simulink model "Projecto"  (R2018a)
settings: Solver=ode4  StartTime=0.0  StopTime=2  FixedStep=5e-6  RelTol=1e-3
values from neighbouring files (symbols this model uses):
  fn = 60    [parametros_motor.m]
  J = 0.089    [parametros_motor.m]
  Llr = 0.002    [parametros_motor.m]
  Lls = 0.002    [parametros_motor.m]
  Pn = 2130    [parametros_motor.m]
  pp = 2    [parametros_motor.m]
  ref_flux = 0.6    [parametros_motor.m]
  ref_vel = 500    [parametros_motor.m]
  Rr = 0.816    [parametros_motor.m]
  Rs = 0.435    [parametros_motor.m]
  Tload = 10    [parametros_motor.m]
  Vdc = 500    [parametros_motor.m]
  Vn = 220    [parametros_motor.m]
undefined symbols (not defined in the file or in its folder): gcbh, pe_sli_rtmsupport
libraries: powerlib x12, powerlib_meascontrol x4, fuzblock x1, spsDrivesSpeedControllerModel x1
settings Model: Creator=up201604509  LastModifiedBy=up201604509
settings SolverCC: ZeroCrossAlgorithm=Adaptive  AlgebraicLoopSolver=LineSearch
settings DebuggingCC: AlgebraicLoopMsg=none  MaxConsecutiveZCsMsg=none

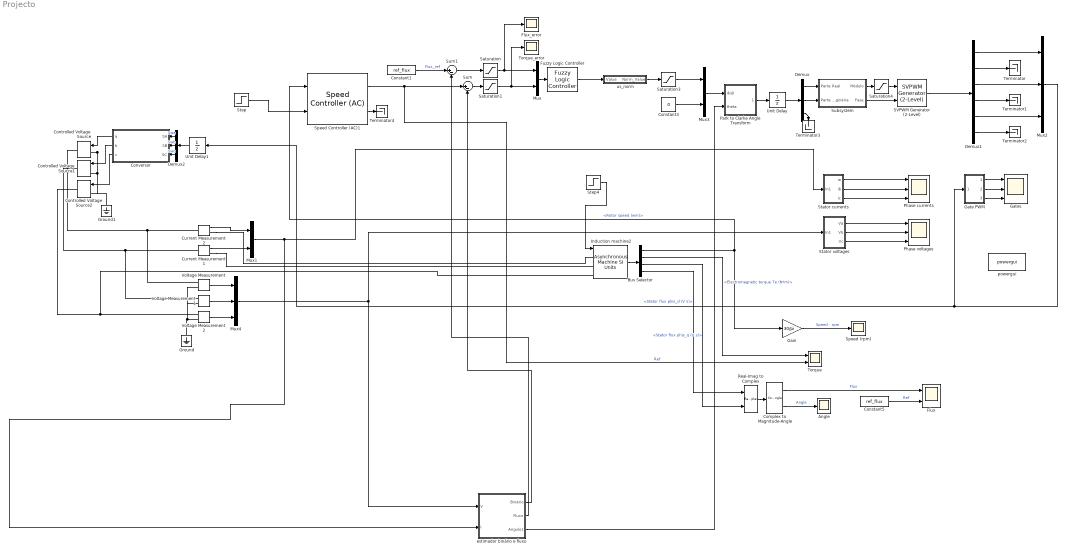
== system Projecto ==
  Angle : Scope
  Bus Selector : BusSelector  OutputSignals=Mechanical.Rotor speed (wm),Mechanical.Electromagnetic torque Te (N*m),Stator measurements.Stator flux phis_q (V s),Stator measurements.Stator flux phis_d (V s)
  Complex to Magnitude-Angle : ComplexToMagnitudeAngle
  Constant1 : Constant  Value=ref_flux
  Constant3 : Constant  Value=0
  Constant5 : Constant  Value=ref_flux
  Controlled Voltage Source : powerlib/Electrical Sources/Controlled Voltage Source  Initialize=on  Source_Type=AC  Amplitude=0  Phase=0  Frequency=0  Measurements=Voltage
      settings: SourceProductName=Simscape Electrical
  Controlled Voltage Source1 : powerlib/Electrical Sources/Controlled Voltage Source  Initialize=on  Source_Type=AC  Amplitude=0  Phase=0  Frequency=0  Measurements=Voltage
      settings: SourceProductName=Simscape Electrical
  Controlled Voltage Source2 : powerlib/Electrical Sources/Controlled Voltage Source  Initialize=on  Source_Type=AC  Amplitude=0  Phase=0  Frequency=0  Measurements=Voltage
      settings: SourceProductName=Simscape Electrical
  Conversor : Subsystem
  Current Measurement1 : powerlib/Measurements/Current Measurement  Tag=PoWeRsYsTeMmEaSuReMeNt  PhasorSimulation=off  OutputType=Complex  PSBequivalent=0
      settings: SourceProductName=Simscape Electrical
  Current Measurement2 : powerlib/Measurements/Current Measurement  Tag=PoWeRsYsTeMmEaSuReMeNt  PhasorSimulation=off  OutputType=Complex  PSBequivalent=0
      settings: SourceProductName=Simscape Electrical
  Demux : Demux  Outputs=3
  Demux1 : Demux  Outputs=6
  Demux2 : Demux  Outputs=3
  Flux : Scope  NumInputPorts=2
  Flux_error : Scope
  Fuzzy Logic Controller : fuzblock/Fuzzy Logic  Controller  FIS=controler  OutputSampleNumber=101  DataType=double  FuzzifiedInputs=off  RuleFiringStrengths=off  RuleOutputs=off  AggregatedOutputs=off  SimulateUsing=Interpreted execution  OutOfRangeInputValueMessage=warning  NoRuleFiredMessage=warning  EmptyOutputFuzzySetMessage=warning
  Gain : Gain  Gain=30/pi  SaturateOnIntegerOverflow=on  OutDataTypeStr=Inherit: Same as input  ParamDataTypeStr=Inherit: Same as input
  Gate PWM : Subsystem
  Gates : Scope  NumInputPorts=3
  Ground : powerlib/Elements/Ground  LConnTagsString=a
      settings: SourceProductName=Simscape Electrical
  Ground1 : powerlib/Elements/Ground  LConnTagsString=a
      settings: SourceProductName=Simscape Electrical
  Induction machine2 : powerlib/Machines/Asynchronous Machine SI Units  RotorType=Squirrel-cage  PresetModel=No  MechanicalLoad=Torque Tm  ShowDetailedParameters=on  ReferenceFrame=Stationary  Units=SI  MeasurementBus=off  NominalParameters="[Pn  Vn  fn]"  Stator=[Rs Lls]  Rotor=[Rr Llr]  Cage1=[ 0.022 0.226/377]  Cage2=[ 0.022 0.226/377]  Lm=Lm  Mechanical="[J  0.001 pp]"  PolePairs=2  InitialConditions=[1 0 0 0 0 0 -120 120]  SimulateSaturation=off  Saturation=[0 0;0 0]  LoadFlowParameters=0  TsPowergui=0  TsBlock=-1  IterativeModel=Trapezoidal non iterative  IterativeDiscreteModel=Trapezoidal non iterative  Pmec=0
      settings: SourceProductName=Simscape Electrical
  Mux : Mux  Inputs=2
  Mux1 : Mux  Inputs=2
  Mux2 : Mux  Inputs=3
  Mux3 : Mux  Inputs=2
  Mux4 : Mux  Inputs=3
  Park to Clarke Angle Transform : Subsystem  AncestorBlock=peTransforms/Park to Clarke Angle Transform  LoadFcn=pe_sli_rtmsupport( 'loadfcn', gcbh );  mask(Park to Clarke Angle Transform){AxisAlignment=D-axis}
      mask prompts: AxisAlignment "Phase-a axis alignment:"
      mask help: This block implements an angle transformation from Park coordinates to Clarke coordinates.
      mask init:
      | switch AxisAlignment
      |     case 'Q-axis'
      |         Offset = pi/2;
      |     case 'D-axis'
      |         Offset = 0;
      |     otherwise
      | end
      settings: CopyFcn=pe_sli_rtmsupport( 'copyfcn', gcbh );  DeleteFcn=pe_sli_rtmsupport( 'deletefcn', gcbh );  ModelCloseFcn=pe_sli_rtmsupport( 'modelclosefcn', gcbh );  PostSaveFcn=pe_sli_rtmsupport( 'postsavefcn', gcbh );  PreCopyFcn=pe_sli_rtmsupport( 'precopyfcn', gcbh );  OpenFcn=pe_sli_rtmsupport( 'openfcn', gcbh );  CloseFcn=pe_sli_rtmsupport( 'closefcn', gcbh );  PreDeleteFcn=pe_sli_rtmsupport( 'predeletefcn', gcbh );
      mask Help: web(nesl_help(gcbh))
      mask TypeOptions AxisAlignment: Q-axis | D-axis
      mask Display: pe.mask.drawParkToClarkeAngleTransform();
  Phase currents : Scope  NumInputPorts=3
  Phase voltages : Scope  NumInputPorts=3
  Real-Imag to Complex : RealImagToComplex
  SVPWM Generator (2-Level) : powerlib_meascontrol/Pulse & Signal Generators/SVPWM Generator (2-Level)  InputType=Magnitude-Angle (rad)  SwitchingPattern=Pattern #1  Fc=10000  ParUref=[0.8 -30 60]  Ts=0
      settings: SourceProductName=Simscape Electrical  SourceProductBaseCode=PS
  Saturation : Saturate
  Saturation1 : Saturate  UpperLimit=20  LowerLimit=-20
  Saturation3 : Saturate  UpperLimit=1  LowerLimit=-1
  Saturation4 : Saturate  UpperLimit=1  LowerLimit=0
  Speed (rpm) : Scope
  Speed Controller (AC)1 : spsDrivesSpeedControllerModel/Speed Controller (AC)  ctrlType=Without flux reference output  SwK=Speed regulation  Ts=5e-6  ramp=[-1800,1800]  kp=5  ki=10  fc=100  ctrl_sat=[-60,60]  Tsc=100e-6  fn=60  p=2  nf=0.3
      settings: SourceProductName=The database C:\Users\ak23510\AppData\Roaming\MathWorks\MATLAB\R2017a\slblocks_master.db is locked, or a table in the database is locked. (database is locked)
  Stator currents : Subsystem
  Stator voltages : Subsystem
  Step : Step  Time=0.15  After=ref_vel  SampleTime=0
  Step4 : Step  Time=0.15  After=Tload  SampleTime=0
  Subsystem : Subsystem
  Sum : Sum  Inputs=|+-
  Sum1 : Sum  Inputs=|+-
  Terminator{,1..4} (5 alike) : Terminator
  Torque : Scope  NumInputPorts=2
  Torque_error : Scope
  Unit Delay : UnitDelay  SampleTime=-1  HasFrameUpgradeWarning=on
  Unit Delay1 : UnitDelay  SampleTime=-1  HasFrameUpgradeWarning=on
  Voltage Measurement : powerlib/Measurements/Voltage Measurement  Tag=PoWeRsYsTeMmEaSuReMeNt  PhasorSimulation=off  OutputType=Complex  PSBequivalent=0
      settings: SourceProductName=Simscape Electrical
  Voltage Measurement1 : powerlib/Measurements/Voltage Measurement  Tag=PoWeRsYsTeMmEaSuReMeNt  PhasorSimulation=off  OutputType=Complex  PSBequivalent=0
      settings: SourceProductName=Simscape Electrical
  Voltage Measurement2 : powerlib/Measurements/Voltage Measurement  Tag=PoWeRsYsTeMmEaSuReMeNt  PhasorSimulation=off  OutputType=Complex  PSBequivalent=0
      settings: SourceProductName=Simscape Electrical
  estimador binário e fluxo : Subsystem
  powergui : powerlib/powergui  Priority=1  SimulationMode=Discrete  SampleTime=5e-6  frequency=60  Iterations=50  frequencyindice=60  Pbase=100e6  ErrMax=1e-4  UnitsV=kV  UnitsW=MW  buscounter=0  FunctionMessages=off  echomessages=off  EnableUseOfTLC=off  CurrentSourceSwitches=off  DisableSnubberDevices=off  DisableRonSwitches=off  DisableVfSwitches=off  DisplayEquations=off  AutomaticDiscreteSolvers=off  SolverType=Tustin/Backward Euler (TBE)  Interpol=off  ExternalGateDelay=off  methode=off  Ts=100  x0status=blocks  SPID=off  SwTol=0  HookPort=off  NonlinearTolerance=0  nMaxIteration=15  ContinueOnMaxIteration=off  RestoreLinks=warning  ResistiveCurrentMeasurement=off  Frange=[0:2:500]  Ylog=off  Xlog=on  ShowGrid=off  save=off  variable=ZData  structure=0  ZoomFFT=off  StartTime=0.0  cycles=1  DisplayStyle=1  fundamental=60  FreqAxis=off  MaxFrequency=1000  frequencyindicesteady=1  RmsSteady=1  display=off
      settings: SourceProductName=Simscape Electrical
  us_norm : Subsystem
  wires:
  SVPWM Generator (2-Level)/1 -> Demux1/1
  Demux1/2 -> Terminator/1
  Demux1/4 -> Terminator1/1
  Demux1/6 -> Terminator2/1
  Demux1/1 -> Mux2/1
  Demux1/3 -> Mux2/2
  Demux1/5 -> Mux2/3
  Mux2/1 -> Unit Delay1/1, Gate PWM/1(In1)
  Gain/1 -> Speed (rpm)/1  "Speed - rpm"
  Mux/1 -> Fuzzy Logic Controller/1
  Induction machine2/1 -> Bus Selector/1
  Bus Selector/1 -> Speed Controller (AC)1/1, Gain/1  "<Rotor speed (wm)>"
  Constant1/1 -> Sum1/1  "Flux_ref"
  Sum1/1 -> Saturation/1
  Sum/1 -> Saturation1/1
  Saturation/1 -> Flux_error/1, Mux/1
  Saturation1/1 -> Torque_error/1, Mux/2
  Bus Selector/2 -> Torque/1  "<Electromagnetic torque Te (N*m)>"
  Speed Controller (AC)1/1 -> Sum/1, Torque/2  "Ref"
  Real-Imag to Complex/1 -> Complex to Magnitude-Angle/1
  estimador binário e fluxo/1("Binário ") -> Sum/2
  estimador binário e fluxo/2(Fluxo) -> Sum1/2
  Complex to Magnitude-Angle/1 -> Flux/1  "Flux"
  estimador binário e fluxo/3(Angulo1) -> Park to Clarke Angle Transform/2(theta)
  Mux3/1 -> Park to Clarke Angle Transform/1(dq0)
  Park to Clarke Angle Transform/1(AlphaBeta0) -> Unit Delay/1
  Complex to Magnitude-Angle/2 -> Angle/1  "Angle"
  Constant3/1 -> Mux3/2
  Saturation3/1 -> Mux3/1
  Fuzzy Logic Controller/1 -> us_norm/1(Value)
  us_norm/1(Norm_Value) -> Saturation3/1
  Stator currents/1(ia) -> Phase currents/1
  Stator currents/2(ib) -> Phase currents/2
  Stator currents/3(ic) -> Phase currents/3
  Gate PWM/1(Swa) -> Gates/1
  Gate PWM/2(Swb) -> Gates/2
  Gate PWM/3(Swc) -> Gates/3
  Stator voltages/1(Va) -> Phase voltages/1
  Stator voltages/2(Vb) -> Phase voltages/2
  Stator voltages/3(Vc) -> Phase voltages/3
  Bus Selector/3 -> Real-Imag to Complex/2  "<Stator flux phis_q (V s)>"
  Bus Selector/4 -> Real-Imag to Complex/1  "<Stator flux phis_d (V s)>"
  Speed Controller (AC)1/2 -> Terminator4/1
  Constant5/1 -> Flux/2  "Ref"
  Step/1 -> Speed Controller (AC)1/2
  Demux2/3 -> Conversor/3(SC)  "Swc"
  Conversor/1(a) -> Controlled Voltage Source/1
  Conversor/2(b) -> Controlled Voltage Source1/1
  Demux2/2 -> Conversor/2(SB)  "Swb"
  Conversor/3(c) -> Controlled Voltage Source2/1
  Demux2/1 -> Conversor/1(SA)  "Swa"
  Unit Delay1/1 -> Demux2/1
  Saturation4/1 -> SVPWM Generator (2-Level)/1
  Subsystem/1(Módulo) -> Saturation4/1
  Demux/2 -> Subsystem/2(Parte Imaginária)
  Demux/3 -> Terminator3/1
  Subsystem/2(Fase) -> SVPWM Generator (2-Level)/2
  Demux/1 -> Subsystem/1(Parte Real)
  Unit Delay/1 -> Demux/1
  Current Measurement2/1 -> Mux1/1
  Current Measurement1/1 -> Mux1/2
  Voltage Measurement/1 -> Mux4/1
  Voltage Measurement1/1 -> Mux4/2
  Voltage Measurement2/1 -> Mux4/3
  Mux4/1 -> estimador binário e fluxo/1(V), Stator voltages/1(In1)
  Mux1/1 -> estimador binário e fluxo/2(I), Stator currents/1(In1)
  Step4/1 -> Induction machine2/1
  connections:
  Current Measurement2/RConn1 -- Induction machine2/LConn1
  Controlled Voltage Source/LConn1 -- Ground1/LConn1 -- Controlled Voltage Source2/LConn1 -- Controlled Voltage Source1/LConn1
  Controlled Voltage Source2/RConn1 -- Induction machine2/LConn3 -- Voltage Measurement2/LConn1
  Current Measurement1/LConn1 -- Voltage Measurement1/LConn1 -- Controlled Voltage Source1/RConn1
  Controlled Voltage Source/RConn1 -- Voltage Measurement/LConn1 -- Current Measurement2/LConn1
  Voltage Measurement2/LConn2 -- Voltage Measurement/LConn2 -- Voltage Measurement1/LConn2 -- Ground/LConn1
  Current Measurement1/RConn1 -- Induction machine2/LConn2

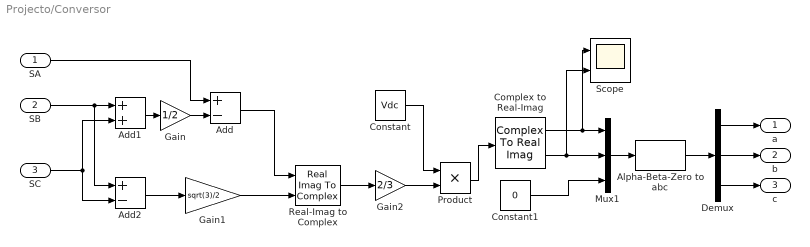
== system Projecto/Conversor ==
  SA : Inport
  SB : Inport  Port=2
  SC : Inport  Port=3
  Add : Sum  Inputs=+-
  Add1 : Sum
  Add2 : Sum  Inputs=+-
  Alpha-Beta-Zero to abc : powerlib_meascontrol/Transformations/Alpha-Beta-Zero to abc
      settings: SourceProductName=Simscape Electrical  SourceProductBaseCode=PS
  Complex to Real-Imag : ComplexToRealImag
  Constant : Constant  Value=Vdc
  Constant1 : Constant  Value=0
  Demux : Demux  Outputs=3
  Gain : Gain  Gain=1/2
  Gain1 : Gain  Gain=sqrt(3)/2
  Gain2 : Gain  Gain=2/3
  Mux1 : Mux  Inputs=3
  Product : Product
  Real-Imag to Complex : RealImagToComplex
  Scope : Scope  NumInputPorts=2
  a : Outport
  b : Outport  Port=2
  c : Outport  Port=3
  wires:
  SA/1 -> Add/1
  SB/1 -> Add2/1, Add1/1
  SC/1 -> Add2/2, Add1/2
  Add1/1 -> Gain/1
  Gain/1 -> Add/2
  Add2/1 -> Gain1/1
  Gain1/1 -> Real-Imag to Complex/2
  Add/1 -> Real-Imag to Complex/1
  Real-Imag to Complex/1 -> Gain2/1
  Gain2/1 -> Product/2
  Constant/1 -> Product/1
  Product/1 -> Complex to Real-Imag/1
  Demux/3 -> c/1
  Demux/2 -> b/1
  Demux/1 -> a/1
  Complex to Real-Imag/1 -> Scope/1, Mux1/1
  Complex to Real-Imag/2 -> Mux1/2, Scope/2
  Constant1/1 -> Mux1/3
  Alpha-Beta-Zero to abc/1 -> Demux/1
  Mux1/1 -> Alpha-Beta-Zero to abc/1

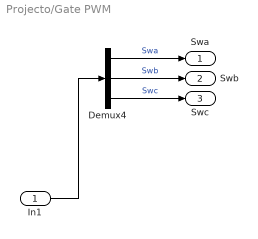
== system Projecto/Gate PWM ==
  In1 : Inport
  Demux4 : Demux  Outputs=3
  Swa : Outport
  Swb : Outport  Port=2
  Swc : Outport  Port=3
  wires:
  Demux4/1 -> Swa/1  "Swa"
  Demux4/2 -> Swb/1  "Swb"
  Demux4/3 -> Swc/1  "Swc"
  In1/1 -> Demux4/1

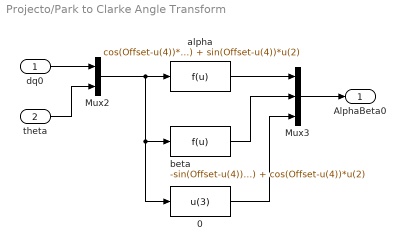
== system Projecto/Park to Clarke Angle Transform ==
  dq0 : Inport
  theta : Inport  Port=2
  0 : Fcn  Expr=u(3)
  Mux2 : Mux  Inputs=2
  Mux3 : Mux  Inputs=3
  alpha : Fcn  Expr=cos(Offset-u(4))*u(1) + sin(Offset-u(4))*u(2)
  beta : Fcn  Expr=-sin(Offset-u(4))*u(1) + cos(Offset-u(4))*u(2)
  AlphaBeta0 : Outport
  wires:
  theta/1 -> Mux2/2
  dq0/1 -> Mux2/1
  Mux2/1 -> 0/1, beta/1, alpha/1
  0/1 -> Mux3/3
  beta/1 -> Mux3/2
  Mux3/1 -> AlphaBeta0/1
  alpha/1 -> Mux3/1

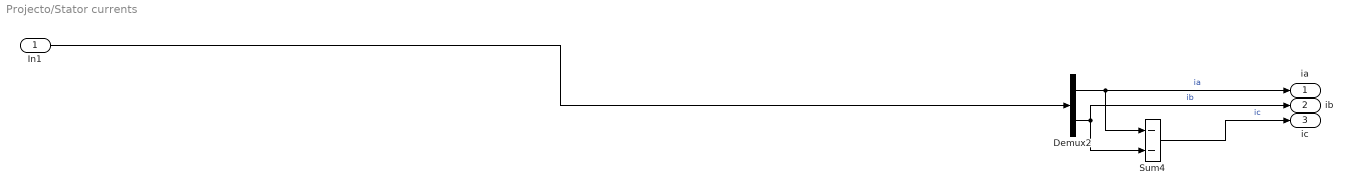
== system Projecto/Stator currents ==
  In1 : Inport
  Demux2 : Demux  Outputs=2
  Sum4 : Sum  Inputs=--  SaturateOnIntegerOverflow=on  InputSameDT=on  OutDataTypeStr=Inherit: Same as first input
  ia : Outport
  ib : Outport  Port=2
  ic : Outport  Port=3
  wires:
  In1/1 -> Demux2/1
  Demux2/1 -> ia/1, Sum4/1  "ia"
  Demux2/2 -> ib/1, Sum4/2  "ib"
  Sum4/1 -> ic/1  "ic"

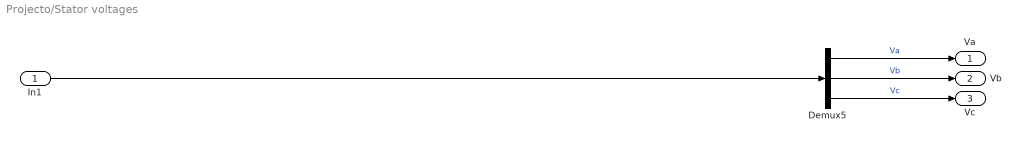
== system Projecto/Stator voltages ==
  In1 : Inport
  Demux5 : Demux  Outputs=3
  Va : Outport
  Vb : Outport  Port=2
  Vc : Outport  Port=3
  wires:
  Demux5/2 -> Vb/1  "Vb"
  In1/1 -> Demux5/1
  Demux5/3 -> Vc/1  "Vc"
  Demux5/1 -> Va/1  "Va"

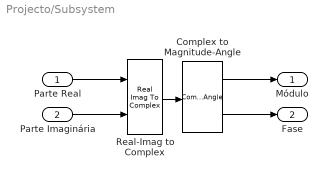
== system Projecto/Subsystem ==
  Parte Real : Inport
  Parte Imaginária : Inport  Port=2
  Complex to Magnitude-Angle : ComplexToMagnitudeAngle
  Real-Imag to Complex : RealImagToComplex
  Módulo : Outport
  Fase : Outport  Port=2
  wires:
  Real-Imag to Complex/1 -> Complex to Magnitude-Angle/1
  Parte Real/1 -> Real-Imag to Complex/1
  Parte Imaginária/1 -> Real-Imag to Complex/2
  Complex to Magnitude-Angle/2 -> Fase/1
  Complex to Magnitude-Angle/1 -> Módulo/1

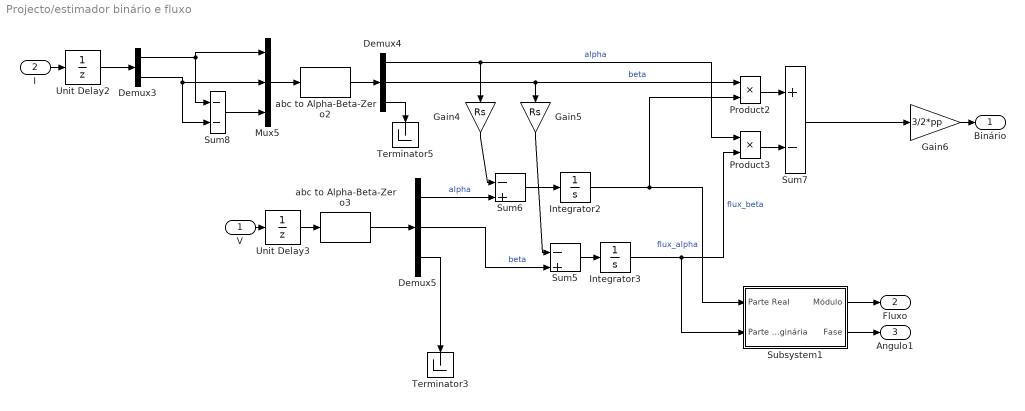
== system Projecto/estimador binário e fluxo ==
  V : Inport
  I : Inport  Port=2
  Demux3 : Demux  Outputs=2
  Demux4 : Demux  Outputs=3
  Demux5 : Demux  Outputs=3
  Gain4 : Gain  Gain=Rs  SaturateOnIntegerOverflow=on  OutDataTypeStr=Inherit: Same as input  ParamDataTypeStr=Inherit: Same as input
  Gain5 : Gain  Gain=Rs  SaturateOnIntegerOverflow=on  OutDataTypeStr=Inherit: Same as input  ParamDataTypeStr=Inherit: Same as input
  Gain6 : Gain  Gain=3/2*pp  SaturateOnIntegerOverflow=on  OutDataTypeStr=Inherit: Same as input  ParamDataTypeStr=Inherit: Same as input
  Integrator2 : Integrator
  Integrator3 : Integrator
  Mux5 : Mux  Inputs=3
  Product2 : Product  SaturateOnIntegerOverflow=on  OutDataTypeStr=Inherit: Same as first input
  Product3 : Product  SaturateOnIntegerOverflow=on  OutDataTypeStr=Inherit: Same as first input
  Subsystem1 : Subsystem
  Sum5 : Sum  Inputs=|-+  SaturateOnIntegerOverflow=on
  Sum6 : Sum  Inputs=|-+  SaturateOnIntegerOverflow=on
  Sum7 : Sum  Inputs=+-  SaturateOnIntegerOverflow=on
  Sum8 : Sum  Inputs=--  SaturateOnIntegerOverflow=on  InputSameDT=on  OutDataTypeStr=Inherit: Same as first input
  Terminator3 : Terminator
  Terminator5 : Terminator
  Unit Delay2 : UnitDelay  SampleTime=-1  HasFrameUpgradeWarning=on
  Unit Delay3 : UnitDelay  SampleTime=-1  HasFrameUpgradeWarning=on
  abc to Alpha-Beta-Zero2 : powerlib_meascontrol/Transformations/abc to Alpha-Beta-Zero
      settings: SourceProductName=Simscape Electrical
  abc to Alpha-Beta-Zero3 : powerlib_meascontrol/Transformations/abc to Alpha-Beta-Zero
      settings: SourceProductName=Simscape Electrical
  "Binário " : Outport
  Fluxo : Outport  Port=2
  Angulo1 : Outport  Port=3
  wires:
  Demux4/1 -> Gain4/1, Product3/1  "alpha"
  Unit Delay2/1 -> Demux3/1
  Sum8/1 -> Mux5/3
  Gain5/1 -> Sum5/1
  Demux5/3 -> Terminator3/1
  Demux4/2 -> Gain5/1, Product2/1  "beta"
  Integrator3/1 -> Subsystem1/2(Parte Imaginária), Product3/2  "flux_beta"
  Unit Delay3/1 -> abc to Alpha-Beta-Zero3/1
  Demux5/2 -> Sum5/2  "beta"
  Sum6/1 -> Integrator2/1
  Integrator2/1 -> Product2/2, Subsystem1/1(Parte Real)  "flux_alpha"
  Sum7/1 -> Gain6/1
  Demux3/1 -> Mux5/1, Sum8/1
  Product3/1 -> Sum7/2
  Sum5/1 -> Integrator3/1
  Mux5/1 -> abc to Alpha-Beta-Zero2/1
  Demux3/2 -> Sum8/2, Mux5/2
  abc to Alpha-Beta-Zero3/1 -> Demux5/1
  abc to Alpha-Beta-Zero2/1 -> Demux4/1
  Product2/1 -> Sum7/1
  Demux4/3 -> Terminator5/1
  Demux5/1 -> Sum6/2  "alpha"
  Gain4/1 -> Sum6/1
  V/1 -> Unit Delay3/1
  I/1 -> Unit Delay2/1
  Subsystem1/1(Módulo) -> Fluxo/1
  Subsystem1/2(Fase) -> Angulo1/1
  Gain6/1 -> "Binário "/1

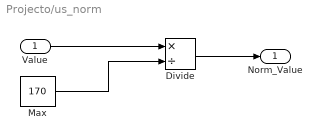
== system Projecto/us_norm ==
  Value : Inport
  Divide : Product  Inputs=*/
  Max : Constant  Value=170
  Norm_Value : Outport
  wires:
  Divide/1 -> Norm_Value/1
  Value/1 -> Divide/1
  Max/1 -> Divide/2

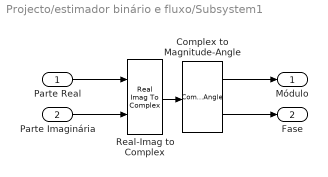
== system Projecto/estimador binário e fluxo/Subsystem1 ==
  Parte Real : Inport
  Parte Imaginária : Inport  Port=2
  Complex to Magnitude-Angle : ComplexToMagnitudeAngle
  Real-Imag to Complex : RealImagToComplex
  Módulo : Outport
  Fase : Outport  Port=2
  wires:
  Real-Imag to Complex/1 -> Complex to Magnitude-Angle/1
  Parte Real/1 -> Real-Imag to Complex/1
  Parte Imaginária/1 -> Real-Imag to Complex/2
  Complex to Magnitude-Angle/2 -> Fase/1
  Complex to Magnitude-Angle/1 -> Módulo/1
